simulink model "complex_test"  (R2019b)
settings: Solver=VariableStepAuto  StartTime=0.0  StopTime=10.0  RelTol=1e-3
values from neighbouring files (symbols this model uses):
  Ac = [real(A) -imag(A);imag(A) real(A)]    [DAC_UIO_Comp.m]    (also in LinearND_QUANTUM_2020_11_14_2.m = [realA -imagA;imagA realA]; UIO_alternative_2021_01_26.m; UIO_alternative_PAPER_2021_02_17.m = Abar(2:3,2:3); UIO_alternative_PAPER_2021_03_01.m = Abar(2:3,2:3))
  imagIC = imag(x0)    [LinearND_QUANTUM_2020_11_14_2.m]
  realIC = real(x0)    [LinearND_QUANTUM_2020_11_14_2.m]
settings Model: Creator=Tris  LastModifiedBy=Tris

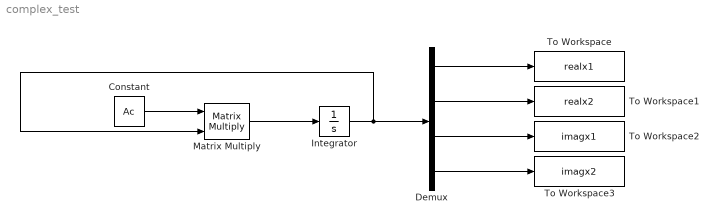
== system complex_test ==
  Constant : Constant  Value=Ac
  Demux : Demux
  Integrator : Integrator  InitialCondition=[realIC;imagIC]
  Matrix Multiply : Product  Multiplication=Matrix(*)
  To Workspace : ToWorkspace  VariableName=realx1  SaveFormat=Timeseries  SampleTime=-1
  To Workspace1 : ToWorkspace  VariableName=realx2  SaveFormat=Timeseries  SampleTime=-1
  To Workspace2 : ToWorkspace  VariableName=imagx1  SaveFormat=Timeseries  SampleTime=-1
  To Workspace3 : ToWorkspace  VariableName=imagx2  SaveFormat=Timeseries  SampleTime=-1
  wires:
  Constant/1 -> Matrix Multiply/1
  Matrix Multiply/1 -> Integrator/1
  Integrator/1 -> Demux/1, Matrix Multiply/2
  Demux/1 -> To Workspace/1
  Demux/2 -> To Workspace1/1
  Demux/3 -> To Workspace2/1
  Demux/4 -> To Workspace3/1
